simulink model "discrete_linear_kalman"  (R2015b)
settings: Solver=VariableStepAuto  StartTime=0.0  StopTime=10.0  RelTol=1e-3
settings Model: Creator=mgreiff  LastModifiedBy=mgreiff

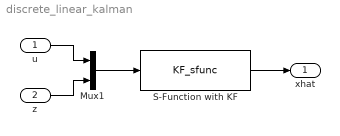
== system discrete_linear_kalman ==
  u : Inport  PortDimensions=KFparam.nControlsignals
  z : Inport  Port=2  PortDimensions=KFparam.nMeasuredStates
  Mux1 : Mux  Inputs=2
  S-Function with KF : S-Function  FunctionName=KF_sfunc  Parameters=KFparam  SFunctionDeploymentMode=off  EnableBusSupport=off
  xhat : Outport
  wires:
  u/1 -> Mux1/1
  z/1 -> Mux1/2
  S-Function with KF/1 -> xhat/1
  Mux1/1 -> S-Function with KF/1
